simulink model "lab5"  (R2016a)
settings: Solver=VariableStepAuto  StartTime=0.0  StopTime=50  RelTol=1e-3
settings Model: Creator=farnamadelkhani  LastModifiedBy=farnamadelkhani

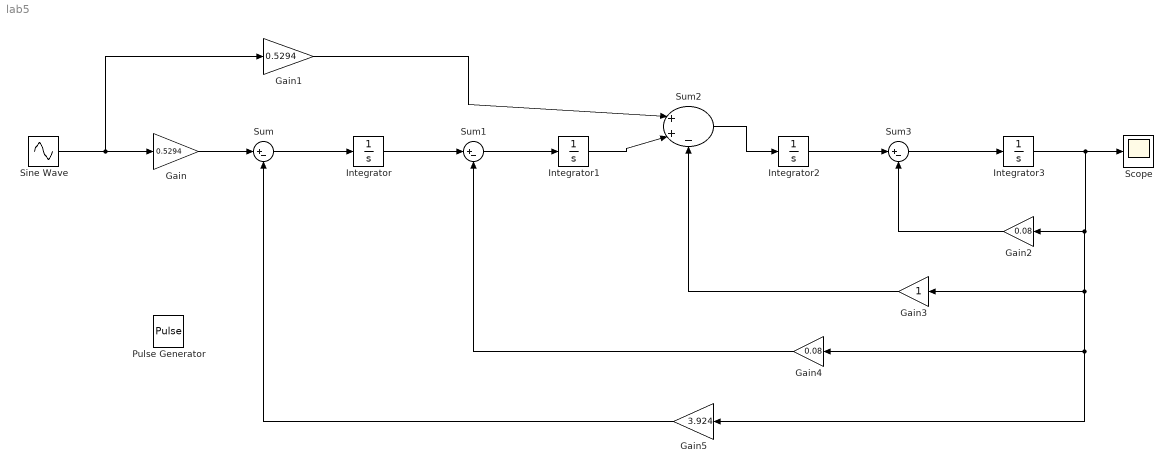
== system lab5 ==
  Gain : Gain  Gain=0.5294
  Gain1 : Gain  Gain=0.5294
  Gain2 : Gain  Gain=0.08
  Gain3 : Gain
  Gain4 : Gain  Gain=0.08
  Gain5 : Gain  Gain=3.924
  Integrator{,1..3} (4 alike) : Integrator
  Pulse Generator : DiscretePulseGenerator  PulseType=Time based  Amplitude=200  Period=10  PulseWidth=.1
  Scope : Scope
  Sine Wave : Sin  Amplitude=200  Frequency=.1  SampleTime=0
  Sum : Sum  Inputs=|+-
  Sum1 : Sum  Inputs=|+-
  Sum2 : Sum  Inputs=|++-
  Sum3 : Sum  Inputs=|+-
  wires:
  Gain/1 -> Sum/1
  Sum/1 -> Integrator/1
  Integrator/1 -> Sum1/1
  Sum1/1 -> Integrator1/1
  Integrator1/1 -> Sum2/2
  Sum2/1 -> Integrator2/1
  Integrator2/1 -> Sum3/1
  Sum3/1 -> Integrator3/1
  Gain1/1 -> Sum2/1
  Integrator3/1 -> Gain2/1, Gain3/1, Gain5/1, Gain4/1, Scope/1
  Gain2/1 -> Sum3/2
  Gain3/1 -> Sum2/3
  Gain4/1 -> Sum1/2
  Gain5/1 -> Sum/2
  Sine Wave/1 -> Gain1/1, Gain/1
